simulink model "acceleration_lqr_controller"  (R2020b)
settings: Solver=VariableStepAuto  StartTime=0.0  StopTime=10.0  RelTol=5e-3
values from neighbouring files (symbols this model uses):
  acceleration_bc = [zeros(6,1), zeros(6,1), zeros(6,1), A, zeros(6,1), zeros(6,1)]    [run_sim.m]
  C_acc = [1,0,0,0,0,0,0,0,0,0,0,0 ... (first row only)    [run_sim.m]
  C_attitude = [1,0,0,0,0,0 ... (first row only)    [run_sim.m]
  inertia = [0.0092, 0, 0 ... (first row only)    [run_sim.m]    (also in symbolic_equations.m = [Ixx, 0, 0)
  J_prop = 0.3    [run_sim.m]
  k = 20    [run_sim.m]
  K_acc = lqr(A_acc, B_acc, Q_acc, R_acc)    [run_sim.m]
  K_attitude = lqr(A_attitude, B_attitude, Q_att, R_att)    [run_sim.m]
  k_r_acc = -inv(C_acc/(A_acc-B_acc*K_acc)*B_acc)    [run_sim.m]
  k_r_attitude = -inv(C_attitude/(A_attitude-B_attitude*K_attitude)*B_attitude)    [run_sim.m]
  l_l = 0.154    [run_sim.m]
  l_s = 0.19    [run_sim.m]
  lambda = 0.01    [run_sim.m]
  m = 0.736    [run_sim.m]
  mass = [0.736, 0, 0 ... (first row only)    [run_sim.m]    (also in symbolic_equations.m = m*eye(3))
  n = [1, -1, 1, -1]    [run_sim.m]    (also in symbolic_equations.m = [1,-1,1,-1])
  rho = 1.1455    [run_sim.m]
  trajectory = [zeros(6,1), lift_vector, t_p_1, P, t_p_2, final_vector]    [run_sim.m]
  trajectory_time = [0, lift_time, p_1_time, circle_time + T, p_2_time, land_time]    [run_sim.m]
  velocity_bc = [zeros(6,1), zeros(6,1), zeros(6,1), V, zeros(6,1), zeros(6,1)]    [run_sim.m]
  wave = 0    [run_sim.m]
  wing_area = 0.000124    [run_sim.m]
undefined symbols (not defined in the file or in its folder): plane_gains
libraries: simulink x2, robotcorelib x1, dspinverses x1
settings Model: OrderedModelArguments=off  Creator=Peter Guglielmino  LastModifiedBy=Peter Guglielmino

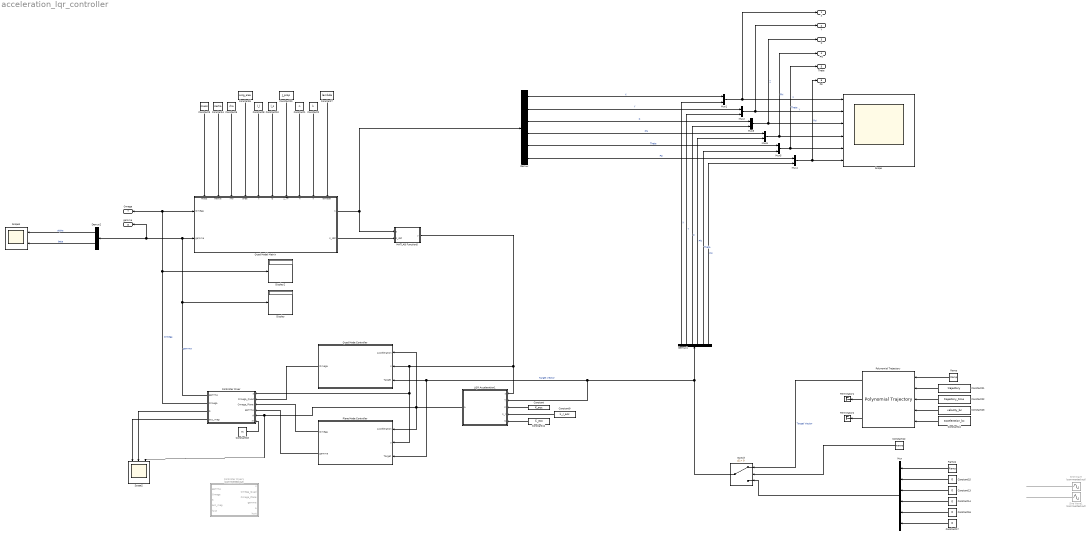
== system acceleration_lqr_controller ==
  Constant : Constant  Value=K_acc
  Constant1 : Constant  Value=n
  Constant10 : Constant  Value=l_s
  Constant11 : Constant  Value=C_acc
  Constant12 : Constant  Value=wave
  Constant{13..17} (5 alike) : Constant  Value=0
  Constant18 : Constant  Value=m
  Constant2 : Constant  Value=k
  Constant20 : Constant  Value=J_prop
  Constant21 : Constant  Value=trajectory
  Constant22 : Constant  Value=trajectory_time
  Constant23 : Constant  Value=velocity_bc
  Constant24 : Constant  Value=acceleration_bc
  Constant3 : Constant  Value=mass
  Constant4 : Constant  Value=inertia
  Constant5 : Constant  Value=rho
  Constant6 : Constant  Value=wing_area
  Constant7 : Constant  Value=lambda
  Constant8 : Constant  Value=l_l
  Constant9 : Constant  Value=k_r_acc
  Controller Mixer : MATLAB Function  TreatAsAtomicUnit=on
  Controller Mixer1 : MATLAB Function  Commented=on  TreatAsAtomicUnit=on
  Demux : Demux  Outputs=6
  Demux1 : Demux  Outputs=6
  Demux2 : Demux  Outputs=2
  Display : Display
  Display2 : Display
  LQR Acceleration1 : MATLAB Function  TreatAsAtomicUnit=on
  MATLAB Function5 : MATLAB Function  TreatAsAtomicUnit=on
  Mux : Mux  Inputs=6
  Mux{1..6} (6 alike) : Mux  Inputs=2
  Plane Mode Controller : Subsystem
  Polynomial Trajectory : robotcorelib/Polynomial Trajectory  WaypointSource=External  Waypoints=[ 0, 2, 1, 5, 0; -1, 3, 1, 4, 4 ]  TimePoints=[ 0, 1, 2, 3, 4 ]  TimeInterval=[ 1, 4 ]  Method=Quintic Polynomial  ParameterSource=External  VelocityBoundaryCondition=zeros( 2, 5 )  AccelerationBoundaryCondition=zeros( 2, 5 )  SimulateUsing=Interpreted execution
  Quad Mode Controller : Subsystem
  Quad Model Matrix : Subsystem
      settings: PortSchema="{\"entries\":[{\"content\":{\"sides\":[{\"content\":{\"connectorIds\":[\"In1\",\"In2\"]},\"type\":\"ConnectorPlacement.EquallySpacedRectSide\",\"uuid\":\"92f3d3d3-fa03-4a7c-b7c8-522e3a278d42\"},{\"content\":{\"connectorIds\":[\"Out1\",\"Out2\"],\"side\":\"RIGHT\"},\"type\":\"ConnectorPlacement.EquallySpacedRectSide\",\"uuid\":\"4b704a1b-c59d-448c-ba8b-d26cf986d8aa\"},{\"content\":{\"connectorIds\":[\"In3\",\"In4\",\"In5\",\"In6\",\"In7\",\"In8\",\"In9\",\"In10\",\"In11\",\"In12\"],\"side\":\"TOP\"},\"type\":\"ConnectorPlacement.EquallySpacedRectSide\",\"uuid\":\"497a2a82-bb5f-47ef-9b21-867d09544019\"},{\"content\":{\"connectorIds\":[],\"side\":\"HIDDEN\"},\"type\":\"ConnectorPlacement.EquallySpacedRectSide\",\"uuid\":\"ae751cc0-2619-44d6-9060-bb188bf8fe67\"}]},\"type\":\"ConnectorPlacement.EquallySpacedConnector\",\"uuid\":\"8022b3ae-a68f-4bf5-ba6d-2aee68313519\"}],\"packageUris\":[\"http://schema.mathworks.com/mf0/Connector/R2020b\"],\"version\":\"1.0\"}"
  Ramp : simulink/Sources/Ramp  slope=0.5  start=0  InitialOutput=0
  Ramp1 : simulink/Sources/Ramp  slope=10  start=0  InitialOutput=0
  Scope : Scope  NumInputPorts=6
  Scope1 : Scope  NumInputPorts=2
  Scope2 : Scope  NumInputPorts=3
  Sine Wave : Sin  Commented=on  Amplitude=0.5  Frequency=2  SampleTime=0
  Sine Wave1 : Sin  Commented=on  Amplitude=0.5  Frequency=2  Phase=pi/2  SampleTime=0
  Switch : Switch  Criteria=u2 > Threshold
  Terminator1 : Terminator
  Terminator2 : Terminator
  X : Outport
  Y : Outport  Port=2
  Z : Outport  Port=3
  Phi : Outport  Port=4
  Theta : Outport  Port=5
  Psi : Outport  Port=6
  Omega : Outport  Port=7
  gamma : Outport  Port=8
  wires:
  Quad Model Matrix/1(s) -> Demux/1, MATLAB Function5/1(s)
  Demux/1 -> Mux1/1  "X"
  Demux/2 -> Mux2/1  "Y"
  Demux/3 -> Mux3/1  "Z"
  Demux/6 -> Mux4/1  "Psi"
  Quad Model Matrix/2(s_dot) -> MATLAB Function5/2(s_dot)
  Demux1/6 -> Mux4/2  "Psi"
  Demux1/1 -> Mux1/2  "X"
  Demux1/3 -> Mux3/2  "Z"
  Demux1/2 -> Mux2/2  "Y"
  Mux1/1 -> Scope/1, X/1  "X"
  Mux2/1 -> Scope/2, Y/1  "Y"
  Mux3/1 -> Z/1, Scope/3  "Z"
  Mux4/1 -> Psi/1, Scope/6  "Psi"
  Constant3/1 -> Quad Model Matrix/3(mass)
  Constant4/1 -> Quad Model Matrix/4(inertia)
  Constant5/1 -> Quad Model Matrix/5(rho)
  Constant6/1 -> Quad Model Matrix/6(area)
  Constant8/1 -> Quad Model Matrix/7(ll)
  Constant10/1 -> Quad Model Matrix/8(ls)
  Constant20/1 -> Quad Model Matrix/9(J_TP)
  Demux1/5 -> Mux5/2  "Theta"
  Demux/5 -> Mux5/1  "Theta"
  Mux5/1 -> Theta/1, Scope/5  "Theta"
  Ramp/1 -> Polynomial Trajectory/1
  Constant22/1 -> Polynomial Trajectory/3
  Constant23/1 -> Polynomial Trajectory/4
  Constant24/1 -> Polynomial Trajectory/5
  Demux1/4 -> Mux6/2  "Phi"
  Polynomial Trajectory/2 -> Terminator1/1
  Polynomial Trajectory/3 -> Terminator2/1
  MATLAB Function5/1(y) -> LQR Acceleration1/1(s), Plane Mode Controller/2(s), Controller Mixer/1(s), Quad Mode Controller/2(s)
  Demux2/1 -> Scope1/1  "alpha"
  Demux2/2 -> Scope1/2  "beta"
  Controller Mixer/1(gamma) -> gamma/1, Demux2/1, Quad Model Matrix/2(gamma), Display/1  "gamma"
  Quad Mode Controller/1(Omega) -> Controller Mixer/2(Omega_Quad)
  Plane Mode Controller/1(Omega) -> Controller Mixer/3(Omega_Plane)
  Plane Mode Controller/2(gamma) -> Controller Mixer/4("gamma ")
  Constant/1 -> LQR Acceleration1/3(K)
  Constant9/1 -> LQR Acceleration1/4(k_r)
  Controller Mixer/2(Omega) -> Omega/1, Quad Model Matrix/1(Omega), Display2/1  "Omega"
  LQR Acceleration1/1(A) -> Quad Mode Controller/1(Acceleration), Plane Mode Controller/1(Acceleration), Scope2/3, Controller Mixer/5(A)
  Constant1/1 -> Quad Model Matrix/10(n)
  Constant2/1 -> Quad Model Matrix/11(k)
  Constant7/1 -> Quad Model Matrix/12(lambda)
  Constant11/1 -> LQR Acceleration1/5(C)
  Mux6/1 -> Phi/1, Scope/4  "Phi"
  Demux/4 -> Mux6/1  "Phi"
  Controller Mixer/3(S) -> Scope2/2
  Controller Mixer/4(acc_mag) -> Scope2/1
  Constant12/1 -> Switch/2
  Constant21/1 -> Polynomial Trajectory/2
  Switch/1 -> Demux1/1, LQR Acceleration1/2(T), Plane Mode Controller/3(Target), Quad Mode Controller/3(Target)  "Target Vector"
  Constant17/1 -> Mux/6
  Constant16/1 -> Mux/5
  Constant14/1 -> Mux/4
  Constant13/1 -> Mux/3
  Mux/1 -> Switch/3
  Constant18/1 -> Controller Mixer/6(m)
  Sine Wave1/1 -> ?
  Sine Wave/1 -> ?
  Ramp1/1 -> Mux/1
  Constant15/1 -> Mux/2
  Polynomial Trajectory/1 -> Switch/1  "Target Vector"

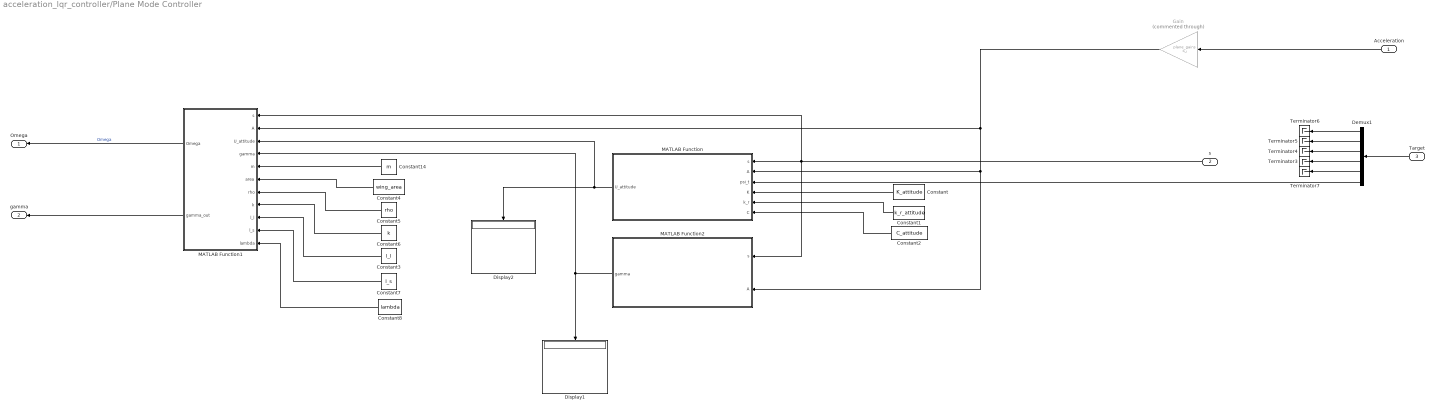
== system acceleration_lqr_controller/Plane Mode Controller ==
  Acceleration : Inport  PortDimensions=[6 1]
  s : Inport  Port=2
  Target : Inport  Port=3
  Constant : Constant  Value=K_attitude
  Constant1 : Constant  Value=k_r_attitude
  Constant14 : Constant  Value=m
  Constant2 : Constant  Value=C_attitude
  Constant3 : Constant  Value=l_l
  Constant4 : Constant  Value=wing_area
  Constant5 : Constant  Value=rho
  Constant6 : Constant  Value=k
  Constant7 : Constant  Value=l_s
  Constant8 : Constant  Value=lambda
  Demux1 : Demux  Outputs=6
  Display1 : Display
  Display2 : Display
  Gain : Gain  Commented=through  Gain=plane_gains  Multiplication=Matrix(K*u)
  MATLAB Function : MATLAB Function  TreatAsAtomicUnit=on
  MATLAB Function1 : MATLAB Function  TreatAsAtomicUnit=on
  MATLAB Function2 : MATLAB Function  TreatAsAtomicUnit=on
  Terminator{3..7} (5 alike) : Terminator
  Omega : Outport
  gamma : Outport  Port=2
  wires:
  MATLAB Function1/1(Omega) -> Omega/1  "Omega"
  Constant14/1 -> MATLAB Function1/5(m)
  MATLAB Function1/2(gamma_out) -> gamma/1
  Constant4/1 -> MATLAB Function1/6(area)
  Constant5/1 -> MATLAB Function1/7(rho)
  Constant6/1 -> MATLAB Function1/8(k)
  s/1 -> MATLAB Function1/1(s), MATLAB Function2/1(s), MATLAB Function/1(s)
  MATLAB Function/1(U_attitude) -> MATLAB Function1/3(U_attitude), Display2/1
  MATLAB Function2/1(gamma) -> MATLAB Function1/4(gamma), Display1/1
  Constant/1 -> MATLAB Function/4(K)
  Constant1/1 -> MATLAB Function/5(k_r)
  Constant2/1 -> MATLAB Function/6(C)
  Constant3/1 -> MATLAB Function1/9(l_l)
  Constant7/1 -> MATLAB Function1/10(l_s)
  Constant8/1 -> MATLAB Function1/11(lambda)
  Demux1/4 -> Terminator3/1
  Demux1/5 -> Terminator7/1
  Target/1 -> Demux1/1
  Demux1/6 -> MATLAB Function/3(psi_t)
  Demux1/2 -> Terminator5/1
  Demux1/3 -> Terminator4/1
  Demux1/1 -> Terminator6/1
  Acceleration/1 -> Gain/1
  Gain/1 -> MATLAB Function1/2(A), MATLAB Function2/2(A), MATLAB Function/2(A)

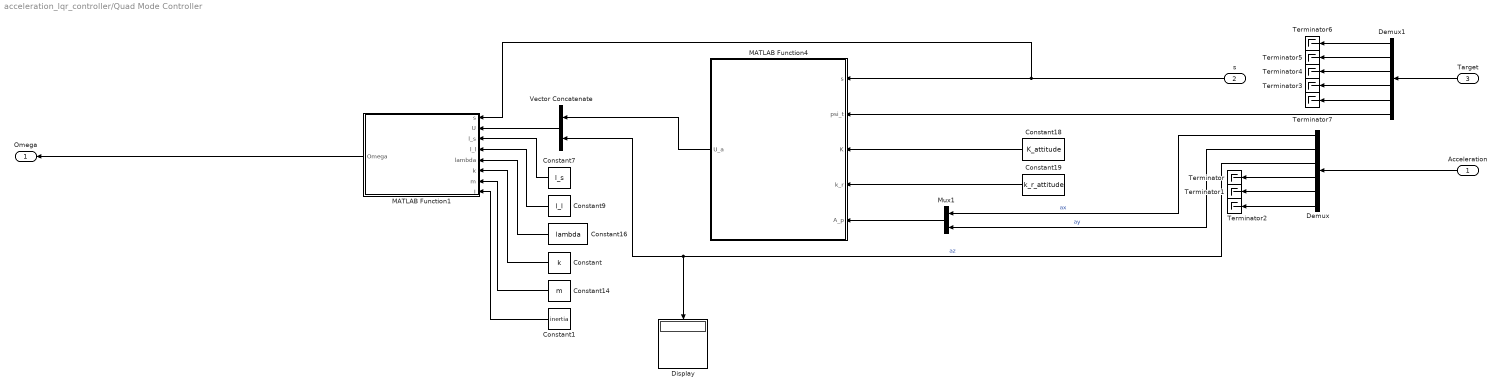
== system acceleration_lqr_controller/Quad Mode Controller ==
  Acceleration : Inport
  s : Inport  Port=2
  Target : Inport  Port=3
  Constant : Constant  Value=k
  Constant1 : Constant  Value=inertia
  Constant14 : Constant  Value=m
  Constant16 : Constant  Value=lambda
  Constant18 : Constant  Value=K_attitude
  Constant19 : Constant  Value=k_r_attitude
  Constant7 : Constant  Value=l_s
  Constant9 : Constant  Value=l_l
  Demux : Demux  Outputs=6
  Demux1 : Demux  Outputs=6
  Display : Display
  MATLAB Function1 : MATLAB Function  TreatAsAtomicUnit=on
  MATLAB Function4 : MATLAB Function  TreatAsAtomicUnit=on
  Mux1 : Mux  Inputs=2
  Terminator{,1..7} (8 alike) : Terminator
  Vector Concatenate : Concatenate
  Omega : Outport
  wires:
  MATLAB Function4/1(U_a) -> Vector Concatenate/1
  Demux/3 -> Vector Concatenate/2, Display/1  "az"
  Constant16/1 -> MATLAB Function1/5(lambda)
  Constant14/1 -> MATLAB Function1/7(m)
  Constant7/1 -> MATLAB Function1/3(l_s)
  Constant9/1 -> MATLAB Function1/4(l_l)
  Constant19/1 -> MATLAB Function4/4(k_r)
  Vector Concatenate/1 -> MATLAB Function1/2(U)
  Constant18/1 -> MATLAB Function4/3(K)
  Demux/4 -> Terminator/1
  Acceleration/1 -> Demux/1
  Demux/1 -> Mux1/1  "ax"
  Demux/2 -> Mux1/2  "ay"
  Mux1/1 -> MATLAB Function4/5(A_p)
  Demux/6 -> Terminator2/1
  Demux/5 -> Terminator1/1
  s/1 -> MATLAB Function1/1(s), MATLAB Function4/1(s)
  Demux1/6 -> MATLAB Function4/2(psi_t)
  Target/1 -> Demux1/1
  Demux1/4 -> Terminator3/1
  Demux1/3 -> Terminator4/1
  Demux1/2 -> Terminator5/1
  Demux1/1 -> Terminator6/1
  Demux1/5 -> Terminator7/1
  Constant/1 -> MATLAB Function1/6(k)
  MATLAB Function1/1(Omega) -> Omega/1
  Constant1/1 -> MATLAB Function1/8(I)

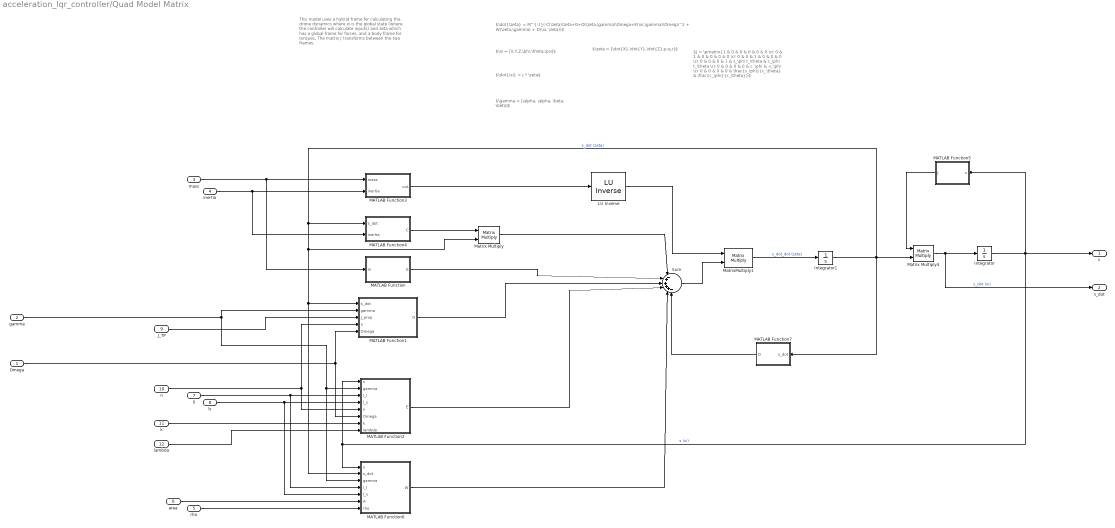
== system acceleration_lqr_controller/Quad Model Matrix ==
  note: This model uses a hybrid frame for calculating the drone dynamics where xi is the global state (where the controller will calculate inputs) and zeta which has a global frame for forces, and a body frame for torques. The matrix J transforms between the two frames.
  note: $\dot{\zeta} = M^{-1}(-C(\zeta)\zeta+G+O(\zeta,\gamma)\Omega+E(\xi,\gamma)\Omega^2 + W(\zeta,\gamma) + D(\xi, \zeta))$
  note: $\gamma = [\alpha, \alpha, \beta, \beta]$
  note: $\xi = [X,Y,Z,\phi,\theta,\psi]$
  note: $\zeta = [\dot{X},\dot{Y},\dot{Z},p,q,r]$
  note: $\dot{\xi} = J * \zeta$
  note: $J = \pmatrix{1 & 0 & 0 & 0 & 0 & 0 \cr 0 & 1 & 0 & 0 & 0 & 0 \cr 0 & 0 & 1 & 0 & 0 & 0 \cr 0 & 0 & 0 & 1 & s_\phi t_\theta & c_\phi t_\theta \cr 0 & 0 & 0 & 0 & c_\phi & -s_\phi \cr 0 & 0 & 0 & 0 & \frac{s_\phi}{c_\theta} & \frac{c_\phi}{c_\theta}}$
  Omega : Inport  PortDimensions=[4,1]
  gamma : Inport  Port=2  PortDimensions=[4 1]
  mass : Inport  Port=3
  inertia : Inport  Port=4
  rho : Inport  Port=5
  area : Inport  Port=6
  ll : Inport  Port=7
  ls : Inport  Port=8
  J_TP : Inport  Port=9
  n : Inport  Port=10
  k : Inport  Port=11
  lambda : Inport  Port=12
  " LU Inverse" : dspinverses/ LU Inverse
  Integrator : Integrator
  Integrator1 : Integrator
  MATLAB Function : MATLAB Function  TreatAsAtomicUnit=on
  MATLAB Function1 : MATLAB Function  TreatAsAtomicUnit=on
  MATLAB Function2 : MATLAB Function  TreatAsAtomicUnit=on
  MATLAB Function3 : MATLAB Function  TreatAsAtomicUnit=on
  MATLAB Function4 : MATLAB Function  TreatAsAtomicUnit=on
  MATLAB Function5 : MATLAB Function  TreatAsAtomicUnit=on
  MATLAB Function6 : MATLAB Function  TreatAsAtomicUnit=on
  MATLAB Function7 : MATLAB Function  TreatAsAtomicUnit=on
  Matrix Multiply : Product  Multiplication=Matrix(*)
  Matrix Multiply4 : Product  Multiplication=Matrix(*)
  MatrixMultiply1 : Product  Multiplication=Matrix(*)
  Sum : Sum  Inputs=|-++++-
  s : Outport
  s_dot : Outport  Port=2
  wires:
  Matrix Multiply/1 -> Sum/1
  rho/1 -> MATLAB Function6/7(rho)
  MatrixMultiply1/1 -> Integrator1/1  "s_dot_dot (zeta)"
  area/1 -> MATLAB Function6/6(A)
  gamma/1 -> MATLAB Function6/3(gamma), MATLAB Function2/2(gamma), MATLAB Function1/2(gamma)
  ll/1 -> MATLAB Function6/4(l_l), MATLAB Function2/3(l_l)
  " LU Inverse"/1 -> MatrixMultiply1/1
  MATLAB Function4/1(C) -> Matrix Multiply/1
  J_TP/1 -> MATLAB Function1/3(J_prop)
  MATLAB Function6/1(W) -> Sum/5
  mass/1 -> MATLAB Function/1(m), MATLAB Function3/1(mass)
  inertia/1 -> MATLAB Function4/2(inertia), MATLAB Function3/2(inertia)
  Sum/1 -> MatrixMultiply1/2
  ls/1 -> MATLAB Function2/4(l_s), MATLAB Function6/5(l_s)
  MATLAB Function2/1(E) -> Sum/4
  MATLAB Function1/1(O) -> Sum/3
  Integrator/1 -> MATLAB Function2/1(s), MATLAB Function6/1(s), s/1, MATLAB Function5/1(s)  "s (xi)"
  MATLAB Function3/1(out) -> " LU Inverse"/1
  MATLAB Function/1(G) -> Sum/2
  Integrator1/1 -> MATLAB Function7/1(s_dot), MATLAB Function4/1(s_dot), Matrix Multiply/2, MATLAB Function6/2(s_dot), MATLAB Function1/1(s_dot), Matrix Multiply4/2  "s_dot (zeta)"
  Omega/1 -> MATLAB Function2/6(Omega), MATLAB Function1/5(Omega)
  MATLAB Function5/1(J) -> Matrix Multiply4/1
  Matrix Multiply4/1 -> s_dot/1, Integrator/1  "s_dot (xi)"
  n/1 -> MATLAB Function2/5(n), MATLAB Function1/4(n)
  k/1 -> MATLAB Function2/7(k)
  lambda/1 -> MATLAB Function2/8(lambda)
  MATLAB Function7/1(D) -> Sum/6

== matlab function acceleration_lqr_controller/Plane Mode Controller/MATLAB Function ==
  data: s input; A input; psi_t input; U_attitude output; K input size=[3 6]; k_r input; C input size=[3 6]
function U_attitude = roll_yaw_control(s, A, psi_t, K, k_r, C)
% This function rolls the drone so that it can line up the rotors with the desired acceleration 

% s = [x, dx, y, dy, z, dz, phi, dphi, theta, dtheta, psi, dpsi]

U_x = A(1);
U_y = A(2);

phi = s(7);
theta = s(9);
psi = s(11);

R = [cos(psi)*cos(theta), -sin(psi)*cos(phi) + cos(psi)*sin(theta)*sin(phi), sin(psi)*sin(phi) + cos(psi)*sin(theta)*cos(phi);
     sin(psi)*cos(theta), cos(psi)*cos(phi) + sin(psi)*sin(theta)*sin(phi), -cos(psi)*sin(phi) + sin(psi)*sin(theta)*cos(phi);
     -sin(theta), cos(theta)*sin(phi), cos(theta)*cos(phi)];

gamma_max = 0.261799;
Kappa_max = sin(gamma_max)^2/(1-sin(gamma_max)^2);
Kappa = min(Kappa_max, U_x^2 + U_y^2);

if (U_x^2 + U_y^2) == 0
    phi_t = 0;
else
    phi_t = -asin(sqrt(Kappa/((1+Kappa)*(U_x^2+U_y^2))) * (U_x*sin(psi) - U_y*cos(psi)));
end

x = s(7:12);

x_d = [phi_t; 0; 0; 0; psi_t; 0];

r = C*x_d;
U_attitude = -K*x + k_r*r;

== matlab function acceleration_lqr_controller/Plane Mode Controller/MATLAB Function2 ==
  data: s input; A input; gamma output
function gamma = tilt_control(s, A)
% This function tilts the rotors to align with the desired acceleration 
% s = [x, dx, y, dy, z, dz, phi, dphi, theta, dtheta, psi, dpsi]

g = 9.8;
m = 0.736;

A = [A(1);
     A(2);
     A(3) - m*g];

phi = s(7);
theta = s(9);
psi = s(11);

R = [cos(psi)*cos(theta), -sin(psi)*cos(phi) + cos(psi)*sin(theta)*sin(phi), sin(psi)*sin(phi) + cos(psi)*sin(theta)*cos(phi);
     sin(psi)*cos(theta), cos(psi)*cos(phi) + sin(psi)*sin(theta)*sin(phi), -cos(psi)*sin(phi) + sin(psi)*sin(theta)*cos(phi);
     -sin(theta), cos(theta)*sin(phi), cos(theta)*cos(phi)];

y_hat = [0; 1; 0]; % Normal vector of the drones x-z plane in the body frame

tilt_vector = R*A - (dot(R*A, y_hat))*y_hat; % Body frame acceleration target projected onto the drones x-z plane 

target_tilt_angle = -atan2(tilt_vector(3), tilt_vector(1));
target_tilt_angle = min(max(target_tilt_angle,-pi/4),5*pi/6);
% target_tilt_angle = pi/2;

gamma = [target_tilt_angle; target_tilt_angle; target_tilt_angle; target_tilt_angle];

== matlab function acceleration_lqr_controller/Quad Mode Controller/MATLAB Function4 ==
  data: s input; psi_t input; U_a output; K input size=[3 6]; k_r input size=[3 3]; A_p input
function U_a  = attitude_control(s, psi_t, K, k_r, A_p)

% s = [x, dx, y, dy, z, dz, phi, dphi, theta, dtheta, psi, dpsi]
% U_p = [U_x, U_y]
% U_x = (cos(phi)*sin(theta)*cos(psi) + sin(phi)*sin(psi))/(cos(phi)*cos(theta))
% U_y = (cos(phi)*sin(theta)*sin(psi) - sin(phi)*cos(psi))/(cos(phi)*cos(theta))
% theta = atan2(U_y + U_x*tan(psi),sin(psi)-cos(psi)^2)
% phi = atan2(U_x*cos(theta)-sin(theta)*cos(psi),sin(psi))
% alpha = pi/2;
% beta = pi/2;

x = s(7:12);

U_x = A_p(1);
U_y = A_p(2);

psi = x(5);

gamma_max = 0.261799;
Kappa_max = sin(gamma_max)^2/(1-sin(gamma_max)^2);
Kappa = min(Kappa_max, U_x^2 + U_y^2);

if (U_x^2 + U_y^2) == 0
    phi = 0;
else
    phi = -asin(sqrt(Kappa/((1+Kappa)*(U_x^2+U_y^2))) * (U_x*sin(psi) - U_y*cos(psi)));
end

s = sign(U_y*sin(psi) + U_x*cos(psi));
inner = 1/(cos(phi)*sqrt(1+Kappa));
inner = min(max(inner,-1),1);
theta = -s*acos(inner);


x_d = [phi; 0; theta; 0; psi_t; 0];
 
C = [1,0,0,0,0,0;
     0,0,1,0,0,0;
     0,0,0,0,1,0];
 
r = C*x_d;
U_a = -K*x + k_r*r;

== matlab function acceleration_lqr_controller/MATLAB Function5 ==
  data: s input; y output; s_dot input
function y = mixer(s, s_dot)

x = [s(1);s_dot(1);s(2);s_dot(2);s(3);s_dot(3);s(4);s_dot(4);s(5);s_dot(5);s(6);s_dot(6)];

y = x;

== matlab function acceleration_lqr_controller/LQR Acceleration1 ==
  data: s input; T input; A output; K input; k_r input; C input
function A = LQR_Acceleration(s, T, K, k_r, C)
% s = [x, dx, y, dy, z, dz, phi, phi_dot, theta, theta_dot, psi, psi_dot]
% T = [x_t, y_t, z_t, phi_t, theta_t, psi_t]

x_t = T(1);
y_t = T(2);
z_t = T(3);
phi_t = T(4);
theta_t = T(5);
psi_t = T(6);

x = s;
x_d = [x_t; 0; y_t; 0; z_t; 0; phi_t; 0; theta_t; 0; psi_t; 0];

r = C*x_d;

A = -K*x + k_r*r;

== matlab function acceleration_lqr_controller/Quad Model Matrix/MATLAB Function6 ==
  data: s input size=[6 1]; s_dot input size=[6 1]; W output size=[6 1]; gamma input size=[4 1]; l_l input; l_s input size=1; A input size=1; rho input size=1
function W = W(s, s_dot, gamma, l_l, l_s, A, rho)
% s_dot = [dx, dy, dz, p, q, r]

phi = s(4);
theta = s(5);
psi = s(6);

R_w = [cos(psi)*cos(theta), -sin(psi)*cos(phi) + cos(psi)*sin(theta)*sin(phi), sin(psi)*sin(phi) + cos(psi)*sin(theta)*cos(phi);
     sin(psi)*cos(theta), cos(psi)*cos(phi) + sin(psi)*sin(theta)*sin(phi), -cos(psi)*sin(phi) + sin(psi)*sin(theta)*cos(phi);
     -sin(theta), cos(theta)*sin(phi), cos(theta)*cos(phi)];

v = R_w*[s_dot(1); s_dot(2); s_dot(3)]; % wind velocity in the direction of the drone

v_x = v(1);
v_z = v(3);
wind_vel = sqrt(v_x^2 + v_z^2);

T = [R_w, zeros(3,3);
     zeros(3,3), eye(3)];

F_w = [0;0;0];
M_w = [0;0;0];

n_x = [1,-1,-1,1]; % Order of lift moment directions in x
n_y = [1,1,-1,-1]; % Order of lift moment directions in y
n_z = [-1,1,-1,1]; % Order of lift moment directions in z

for i = 1:4
    
    attack_angle = atan2(v_z,v_x) - gamma(i);
    F_i = [-1/2*getDragCoef(rad2deg(attack_angle))*rho*A*wind_vel^2;
                                  0;
           -1/2*getLiftCoef(rad2deg(attack_angle))*rho*A*wind_vel^2];
    
    R = getWingR(gamma(i));
    
    F_w = F_w + R*F_i;
    
    M_i = [n_x(i)*l_s*F_i(1);
           n_y(i)*l_l*F_i(2);
           n_z(i)*l_s*F_i(3)];
       
    M_w = M_w + M_i;
end

W = T*[F_w; M_w];

end

function c_l = getLiftCoef(x)
    if x > 0 && x < 90
        c_l = -1E-10*x^6 + 8E-08*x^5 - 2E-06*x^4 + 8E-05*x^3 - 0.0015*x^2 + 0.0329*x + 0.0507;
    else
        c_l = 0;
    end
end

function c_d = getDragCoef(x)
    if x > 0 && x < 90
        c_d = 1E-09*x^5 - 2E-07*x^4 + 3E-06*x^3 - 0.0005*x^2 + 0.0058*x + 0.0456;
    else
        c_d = 0;
    end
end

function R = getWingR(a)
    R = [cos(a), 0, sin(a);
           0,    1,    0;
        -sin(a), 0, cos(a)];
end

== matlab function acceleration_lqr_controller/Plane Mode Controller/MATLAB Function1 ==
  data: s input; A input; U_attitude input size=[3 1]; gamma input; Omega output size=[4 1]; m input; area input; gamma_out output; rho input; k input; l_l input; l_s input; lambda input
function [Omega, gamma_out] = U_to_Omega(s, A, U_attitude, gamma, m, area, rho, k, l_l, l_s, lambda)
% s = [x, dx, y, dy, z, dz, phi, p, theta, q, psi, r]

% Inverse the wing dynamics
x_dot = s(2);
y_dot = s(4);
z_dot = s(6);

phi = s(4);
theta = s(5);
psi = s(6);

R_w = [cos(psi)*cos(theta), -sin(psi)*cos(phi) + cos(psi)*sin(theta)*sin(phi), sin(psi)*sin(phi) + cos(psi)*sin(theta)*cos(phi);
       sin(psi)*cos(theta), cos(psi)*cos(phi) + sin(psi)*sin(theta)*sin(phi), -cos(psi)*sin(phi) + sin(psi)*sin(theta)*cos(phi);
       -sin(theta), cos(theta)*sin(phi), cos(theta)*cos(phi)];

v = R_w*[x_dot; y_dot; z_dot]; % wind velocity in the direction of the drone

v_x = v(1);
v_z = v(3);
wind_vel = sqrt(v_x^2 + v_z^2);

F_w = [0;0;0];

for i = 1:4
    attack_angle = atan2(v_z,v_x) - gamma(i);
    F_i = [-1/2*getDragCoef(rad2deg(attack_angle))*rho*area*wind_vel^2;
                                  0;
           -1/2*getLiftCoef(rad2deg(attack_angle))*rho*area*wind_vel^2];
    
    R = getWingR(gamma(i));
    
    F_w = F_w + R*F_i;
end

g = 9.8;

X_tilde = (m*A(1) - F_w(1));
Y_tilde = (m*A(2) - F_w(2));
Z_tilde = (m*A(3) - F_w(3) - m*g);

U_1 = sqrt(X_tilde^2 + Y_tilde^2 + Z_tilde^2);

% Calculate desired motor thrusts
U_n = [U_1; U_attitude];

U_mat = [k, k, k, k;
        -k*lambda*cos(gamma(1)) + k*l_s*sin(gamma(1)), k*lambda*cos(gamma(2)) - k*l_s*sin(gamma(2)), -k*lambda*cos(gamma(3)) - k*l_s*sin(gamma(3)), k*lambda*cos(gamma(4)) + k*l_s*sin(gamma(4));
         k*l_l*sin(gamma(1)), k*l_l*sin(gamma(2)), -k*l_l*sin(gamma(3)), -k*l_l*sin(gamma(4));
         k*lambda*sin(gamma(1)) + k*l_s*cos(gamma(1)), -k*lambda*sin(gamma(2)) - k*l_s*cos(gamma(2)), k*lambda*sin(gamma(3)) - k*l_s*cos(gamma(3)), -k*lambda*sin(gamma(4)) + k*l_s*cos(gamma(4))];

O_sqr = U_mat\U_n;

if (O_sqr(1) > 0)
    omega_1 = min(sqrt(O_sqr(1)),0.4);
else
    omega_1 = 0;
end

if (O_sqr(2) > 0)
    omega_2 = min(sqrt(O_sqr(2)),0.4);
else
    omega_2 = 0;
end

if (O_sqr(3) > 0)
    omega_3 = min(sqrt(O_sqr(3)),0.4);
else
    omega_3 = 0;
end

if (O_sqr(4) > 0)
    omega_4 = min(sqrt(O_sqr(4)),0.4);
else
    omega_4 = 0;
end

Omega = [omega_1; omega_2; omega_3; omega_4];
gamma_out = gamma;
end

function c_l = getLiftCoef(x)
    if x > 0 && x < 90
        c_l = -1E-10*x^6 + 8E-08*x^5 - 2E-06*x^4 + 8E-05*x^3 - 0.0015*x^2 + 0.0329*x + 0.0507;
    else
        c_l = 0;
    end
end

function c_d = getDragCoef(x)
    if x > 0 && x < 90
        c_d = 1E-09*x^5 - 2E-07*x^4 + 3E-06*x^3 - 0.0005*x^2 + 0.0058*x + 0.0456;
    else
        c_d = 0;
    end
end

function R = getWingR(a)
    R = [cos(a), 0, sin(a);
           0,    1,    0;
        -sin(a), 0, cos(a)];
end

== matlab function acceleration_lqr_controller/Controller Mixer1 ==
  data: s input; Omega_Quad input; gamma output; Omega output; Omega_Plane input; gamma input size=[4 1]; A input; S output; acc_mag output; hyst input boolean; hyst output
function [gamma, Omega, S, acc_mag, hyst] = controller_mixer(s, Omega_Quad, Omega_Plane, gamma, A, hyst)

% This function mixes together the input from the quad mode controller and
% the plane mode controller depending on the angle of the target
% acceleration vector relative to the drones normal vector. These two
% controllers are mixed together with a sigmoid function.

% phi = s(7);
% theta = s(9);
% psi = s(11);
% 
% R = [cos(psi), -sin(psi), 0;
%      sin(psi), cos(psi), 0;
%      0, 0, 1];
% 
% y_hat = [0; 1; 0]; % Normal vector of the drones x-z plane in the body frame
% 
% acceleration_target = R*A(1:3) - (dot(R*A(1:3), y_hat))*y_hat; % Body frame acceleration target projected onto the drones x-z plane 

% acceleration_target_angle = atan2d(acceleration_target(3), acceleration_target(1));

radius = 10;

acc_mag = norm(A(1:3))/radius;

steepness  = 15;
center = 0.5;
band = 0.1;

if isempty(hyst)
    hyst = true;
end

if hyst
    S = 1/(1 + exp(-steepness*(acc_mag - center - band)));
else
    S = 1/(1 + exp(-steepness*(acc_mag - center + band)));
end

if (S > 0.9 && hyst == true)
    hyst = false; 
elseif (S < 0.1 && hyst == false)
    hyst = true;
end

gamma = pi/2 * (1-S) + gamma * S;
Omega = Omega_Quad * (1-S) + Omega_Plane * S;

== matlab function acceleration_lqr_controller/Controller Mixer ==
  data: s input; Omega_Quad input; gamma output; Omega output; Omega_Plane input; gamma input size=[4 1]; A input; S output; acc_mag output; m input
function [gamma, Omega, S, acc_mag] = controller_mixer(s, Omega_Quad, Omega_Plane, gamma, A, m)

% This function mixes together the input from the quad mode controller and
% the plane mode controller depending on the angle of the target
% acceleration vector relative to the drones normal vector. These two
% controllers are mixed together with a sigmoid function.

% phi = s(7);
% theta = s(9);
% psi = s(11);
% 
% R = [cos(psi), -sin(psi), 0;
%      sin(psi), cos(psi), 0;
%      0, 0, 1];
% 
% y_hat = [0; 1; 0]; % Normal vector of the drones x-z plane in the body frame
% 
% acceleration_target = R*A(1:3) - (dot(R*A(1:3), y_hat))*y_hat; % Body frame acceleration target projected onto the drones x-z plane 

% acceleration_target_angle = atan2d(acceleration_target(3), acceleration_target(1));

% g = 9.8;

A_x = A(1);
A_y = A(2);
A_z = A(3);

radius = 5;
acc_mag = norm([A_x, A_y, A_z])/radius;

steepness  = 25;
center = 1;

S = 1/(1 + exp(-steepness*(acc_mag - center)));
% S = 1;

gamma = pi/2 * (1-S) + gamma * S;
Omega = Omega_Quad * (1-S) + Omega_Plane * S;

== matlab function acceleration_lqr_controller/Quad Model Matrix/MATLAB Function1 ==
  data: s_dot input; gamma input size=[4 1]; O output size=[6 1]; J_prop input; n input; Omega input
function O = O(s_dot, gamma, J_prop, n, Omega)
% Gyroscopic force matrix in the body frame
% s_dot = [X_dot, Y_dot, Z_dot, p, q, r] (zeta)

w_b = s_dot(4:6);

gyro = [0;0;0];
for i = 1:4
    gamma_vector = [cos(gamma(i)); 0; -sin(gamma(i))];
    new_vector  = cross(n(i)*w_b, gamma_vector*Omega(i));
    gyro = gyro + new_vector;
end

O = J_prop * [zeros(3,1); gyro];

== matlab function acceleration_lqr_controller/Quad Model Matrix/MATLAB Function ==
  data: m input; G output
function G = G(m)
% Gravity matrix in the world frame
G = m(1)*[0;0;9.8;0;0;0];

== matlab function acceleration_lqr_controller/Quad Model Matrix/MATLAB Function2 ==
  data: s input; E output; gamma input size=[4 1]; l_l input; l_s input; n input; Omega input; k input; lambda input
function E = E(s, gamma, l_l, l_s, n, Omega, k, lambda)
% Thrust force and moment matrix in the hybrid frame
% s = [X, Y, Z, phi, theta, psi] (xi)

phi = s(4);
theta = s(5);
psi = s(6);

% Transformation matrix from the body frame to the world frame
R = [cos(psi)*cos(theta), -sin(psi)*cos(phi) + cos(psi)*sin(theta)*sin(phi), sin(psi)*sin(phi) + cos(psi)*sin(theta)*cos(phi);
     sin(psi)*cos(theta), cos(psi)*cos(phi) + sin(psi)*sin(theta)*sin(phi), -cos(psi)*sin(phi) + sin(psi)*sin(theta)*cos(phi);
     -sin(theta), cos(theta)*sin(phi), cos(theta)*cos(phi)];

% Thrust generated by the spinning motor
Thrust = [k*Omega(1)^2; k*Omega(2)^2; k*Omega(3)^2; k*Omega(4)^2];
 
% Calculate the forces from the thrust in the body frame
F_angles = [cos(gamma(1)), cos(gamma(2)), cos(gamma(3)), cos(gamma(4));
                  0,             0,             0,             0;
            -sin(gamma(1)), -sin(gamma(2)), -sin(gamma(3)), -sin(gamma(4))];
       
F_thrust = F_angles * Thrust;

% Calculate the moments from the thrust in the body frame
M_arms = [l_s*sin(gamma(1)) - lambda*n(1)*cos(gamma(1)), -l_s*sin(gamma(2)) - lambda*n(2)*cos(gamma(2)), -l_s*sin(gamma(3)) - lambda*n(3)*cos(gamma(3)), l_s*sin(gamma(4)) - lambda*n(4)*cos(gamma(4));
          l_l * sin(gamma(1)), l_l * sin(gamma(2)), -l_l * sin(gamma(3)), -l_l * sin(gamma(4));
          l_s*cos(gamma(1)) + lambda*n(1)*sin(gamma(1)), -l_s*cos(gamma(2)) + lambda*n(2)*sin(gamma(2)), -l_s*cos(gamma(3)) + lambda*n(3)*sin(gamma(3)), l_s*cos(gamma(4)) + lambda*n(4)*sin(gamma(4))];

M_thrust = M_arms * Thrust;
      
% Convert the forces and moments to the hybrid frame 
E = [R*F_thrust;
     M_thrust];

== matlab function acceleration_lqr_controller/Quad Model Matrix/MATLAB Function3 ==
  data: mass input; out output; inertia input
function out = M(mass, inertia)
% Mass matrix in the body frame

M = mass * eye(3);

out = [M, zeros(3,3);
    zeros(3,3), inertia];

== matlab function acceleration_lqr_controller/Quad Model Matrix/MATLAB Function4 ==
  data: s_dot input; C output size=[6,6]; inertia input
function C = C(s_dot, inertia)
% Coriolis matrix in the body frame
% s_dot = [X_dot, Y_dot, Z_dot, p, q, r] (zeta)

skew = inertia*s_dot(4:6);

C = [zeros(3,3), zeros(3,3);
     zeros(1,3), 0, skew(3), -skew(2);
     zeros(1,3), -skew(3), 0, skew(1);
     zeros(1,3), skew(2), -skew(1), 0];

== matlab function acceleration_lqr_controller/Quad Model Matrix/MATLAB Function5 ==
  data: s input; J output
function J = J(s)

phi = s(4);
theta = s(5);

J = [1, 0, 0, 0, 0, 0;
     0, 1, 0, 0, 0, 0;
     0, 0, 1, 0, 0, 0;
     0, 0, 0, 1, sin(phi)*tan(theta), cos(phi)*tan(theta);
     0, 0, 0, 0, cos(phi), -sin(phi);
     0, 0, 0, 0, sin(phi)/cos(theta), cos(phi)/cos(theta)];

== matlab function acceleration_lqr_controller/Quad Model Matrix/MATLAB Function7 ==
  data: s_dot input; D output
function D = D(s_dot)

drag_matrix = [0.1,0,0,0,0,0;
               0,0.1,0,0,0,0;
               0,0,0.1,0,0,0;
               0,0,0,0.01,0,0;
               0,0,0,0,0.01,0;
               0,0,0,0,0,0.01];

D = drag_matrix*s_dot.^2;

== matlab function acceleration_lqr_controller/Quad Mode Controller/MATLAB Function1 ==
  data: s input; U input size=4; l_s input; l_l input; lambda input; k input; m input; I input; Omega output
function Omega = U_to_Omega(s, U, l_s, l_l, lambda, k, m, I)

% s = [x, dx, y, dy, z, dz, phi, dphi, theta, dtheta, psi, dpsi]
% U = [U2, U3, U4, Uz]
% U1 = b*(omega_1^2 + omega_2^2 + omega_3^2 + omega_4^2)
% U2 = lb*(-omega_2^2 + omega_4^2)
% U3 = lb*(-omega_1^2 + omega_3^2)
% U4 = d*(-omega_1^2 + omega_2^2 - omega_3^2 + omega_4^2)
% Ux = cos(phi)sin(theta)cos(psi) + sin(phi)cos(psi)
% Uy = cos(phi)sin(theta)sin(psi) - sin(phi)cos(psi)
% Uz = g + (cos(phi)cos(theta))*1/m*U1

phi = s(7);
theta = s(9);

Ixx = I(1);
Iyy = I(5);
Izz = I(9);
g = 9.8;

U_1 = -m*(U(4) - g)/(cos(phi)*cos(theta));

U_n = [U_1; U(1:3)];

U_mat = [k, k, k, k;
         k*l_s, -k*l_s, -k*l_s, k*l_s;
         k*l_l, k*l_l, -k*l_l, -k*l_l;
         k*lambda, -k*lambda, k*lambda, -k*lambda];

O_sqr = U_mat\U_n;

if (O_sqr(1) > 0)
    omega_1 = min(sqrt(O_sqr(1)),0.4);
else
    omega_1 = 0;
end

if (O_sqr(2) > 0)
    omega_2 = min(sqrt(O_sqr(2)),0.4);
else
    omega_2 = 0;
end

if (O_sqr(3) > 0)
    omega_3 = min(sqrt(O_sqr(3)),0.4);
else
    omega_3 = 0;
end

if (O_sqr(4) > 0)
    omega_4 = min(sqrt(O_sqr(4)),0.4);
else
    omega_4 = 0;
end

Omega = [omega_1; omega_2; omega_3; omega_4];
